simulink model "nav_sliding"  (R2022b)
settings: Solver=FixedStepAuto  StartTime=0.0  StopTime=10.0  FixedStep=0.01  RelTol=1e-3
values from neighbouring files (symbols this model uses):
  aR = diag([ar; ap; ay])    [main_flock3.m]    (also in main_flock4.m; main_sliding.m)
  Att_1 = [2 -2 -15]    [main_sliding.m]
  K1 = diag([k111; k122; k133])    [main_flock3.m]    (also in main_flock4.m; main_sliding.m)
  K2 = diag([k211; k222; k233])    [main_flock3.m]    (also in main_flock4.m; main_sliding.m)
  Ki = diag([Ki1; Ki2; Ki3])    [main_flock3.m]    (also in main_flock4.m; main_sliding.m)
  lam = diag([lam1; lam2; lam3])    [main_flock3.m]    (also in main_flock4.m; main_sliding.m)
  X0_1 = [P01 dP01 om01]    [main_flock3.m]    (also in main_flock4.m; main_sliding.m = [P0 dP0 om0])
undefined symbols (not defined in the file or in its folder): A_Euler
libraries: aerosimlib x1
settings Model: Creator=root  LastModifiedBy=jonatan_alvarez
settings SolverCC: AlgebraicLoopSolver=TrustRegion
settings DataIOCC: ReturnWorkspaceOutputs=off
settings DebuggingCC: UnconnectedInputMsg=warning  UnconnectedOutputMsg=warning  UnconnectedLineMsg=warning  SFMachineParentedDataDiag=warning  ArithmeticOperatorsInVariantConditions=warning
settings ModelReferenceCC: EnableRefExpFcnMdlSchedulingChecks=on
settings SFSimCC: CustomCodeUndefinedFunction=UseInterfaceOnly

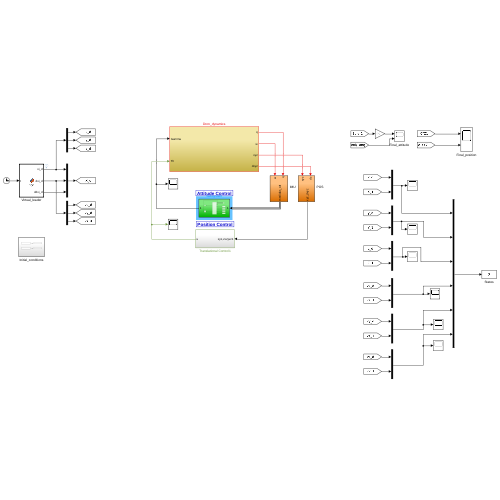
[thumbnail: Simulink's stored preview of the top-level diagram]
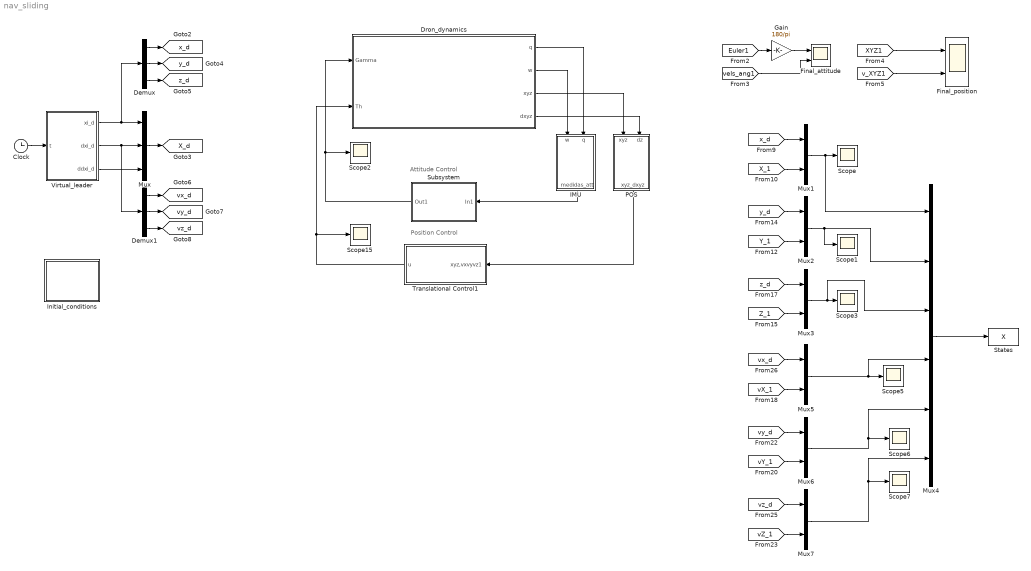
== system nav_sliding ==
  note: Position Control
  note: Attitude Control
  Clock : Clock
  Demux : Demux  Outputs=3
  Demux1 : Demux  Outputs=3
  Dron_dynamics : Subsystem
  Final_attitude : Scope  NumInputPorts=2
  Final_position : Scope  NumInputPorts=2
  Gain : Gain  Gain=180/pi
  "IMU " : Subsystem
  Initial_conditions : Subsystem
  Mux : Mux  Inputs=3
  Mux{1..3,5..7} (6 alike) : Mux  Inputs=2
  Mux4 : Mux  Inputs=6
  "POS " : Subsystem
  Scope{,1..3,5..7,15} (8 alike) : Scope
  States : ToWorkspace  VariableName=X  SampleTime=-1
  Subsystem : Subsystem
  Translational Control1 : Subsystem
  Virtual_leader : MATLAB Function  TreatAsAtomicUnit=on
  tag scope: X_d=global, vx_d=global, vy_d=global, vz_d=global, x_d=global, y_d=global, z_d=global
  wires:
  [vels_ang1] -> Final_attitude/2
  [v_XYZ1] -> Final_position/2
  Gain/1 -> Final_attitude/1
  [XYZ1] -> Final_position/1
  [Euler1] -> Gain/1
  Dron_dynamics/2(w) -> "IMU "/1(w)
  Dron_dynamics/4(dxyz) -> "POS "/2(dz)
  Mux/1 -> [X_d]
  Virtual_leader/3(ddxi_d) -> Mux/3
  Dron_dynamics/1(q) -> "IMU "/2(q)
  Subsystem/1(Out1) -> Scope2/1, Dron_dynamics/1(Gamma)
  Dron_dynamics/3(xyz) -> "POS "/1(xyz)
  "POS "/1(xyz_dxyz) -> Translational Control1/1(xyz,vxvyvz1)
  Translational Control1/1(u) -> Scope15/1, Dron_dynamics/2(Th)
  "IMU "/1(medidas_att) -> Subsystem/1(In1)
  Virtual_leader/1(xi_d) -> Demux/1, Mux/1
  Demux/1 -> [x_d]
  Demux/2 -> [y_d]
  Demux/3 -> [z_d]
  [x_d] -> Mux1/1
  [X_1] -> Mux1/2
  Mux2/1 -> Mux4/2, Scope1/1
  [Y_1] -> Mux2/2
  [y_d] -> Mux2/1
  [z_d] -> Mux3/1
  [Z_1] -> Mux3/2
  Mux3/1 -> Mux4/3, Scope3/1
  Mux4/1 -> States/1
  Mux1/1 -> Mux4/1, Scope/1
  Demux1/3 -> [vz_d]
  Demux1/2 -> [vy_d]
  Demux1/1 -> [vx_d]
  Virtual_leader/2(dxi_d) -> Demux1/1, Mux/2
  [vZ_1] -> Mux7/2
  [vz_d] -> Mux7/1
  [vy_d] -> Mux6/1
  [vY_1] -> Mux6/2
  [vX_1] -> Mux5/2
  [vx_d] -> Mux5/1
  Mux5/1 -> Scope5/1, Mux4/4
  Mux6/1 -> Scope6/1, Mux4/5
  Mux7/1 -> Scope7/1, Mux4/6
  Clock/1 -> Virtual_leader/1(t)

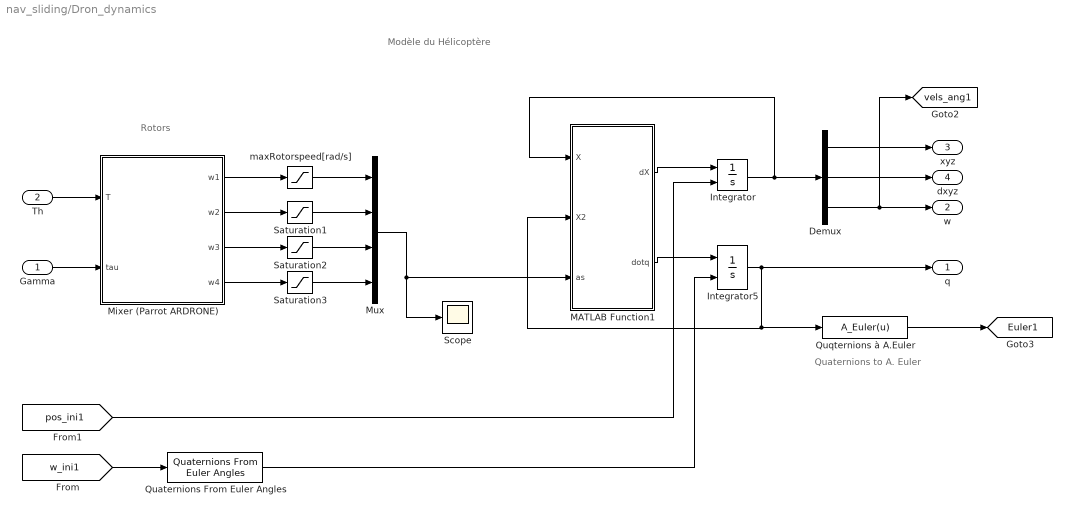
== system nav_sliding/Dron_dynamics ==
  note: Modèle du Hélicoptère
  note: Rotors
  note: Quaternions to A. Euler
  Gamma : Inport
  Th : Inport  Port=2
  Demux : Demux  Outputs=3
  Integrator : Integrator  InitialConditionSource=external
  Integrator5 : Integrator  InitialConditionSource=external  InitialCondition=[1 0 0 0]
  MATLAB Function1 : MATLAB Function  TreatAsAtomicUnit=on
  Mixer (Parrot ARDRONE) : MATLAB Function  TreatAsAtomicUnit=on
  Mux : Mux
  Quaternions From Euler Angles : aerosimlib/Transformations/Quaternions From Euler Angles
  Quqternions à A.Euler : MATLABFcn  MATLABFcn=A_Euler(u)  OutputDimensions=3
  Saturation1 : Saturate  UpperLimit=1100  LowerLimit=5
  Saturation2 : Saturate  UpperLimit=1100  LowerLimit=5
  Saturation3 : Saturate  UpperLimit=1100  LowerLimit=5
  Scope : Scope
  maxRotorspeed[rad/s] : Saturate  UpperLimit=1100  LowerLimit=5
  q : Outport  VectorParamsAs1DForOutWhenUnconnected=off
  w : Outport  Port=2  VectorParamsAs1DForOutWhenUnconnected=off
  xyz : Outport  Port=3  VectorParamsAs1DForOutWhenUnconnected=off
  dxyz : Outport  Port=4  VectorParamsAs1DForOutWhenUnconnected=off
  tag scope: Euler1=global, vels_ang1=global
  wires:
  [w_ini1] -> Quaternions From Euler Angles/1
  Quqternions à A.Euler/1 -> [Euler1]
  Mixer (Parrot ARDRONE)/4(w4) -> Saturation3/1
  Saturation1/1 -> Mux/2
  Mixer (Parrot ARDRONE)/2(w2) -> Saturation1/1
  Mixer (Parrot ARDRONE)/1(w1) -> maxRotorspeed[rad/s]/1
  maxRotorspeed[rad/s]/1 -> Mux/1
  Saturation3/1 -> Mux/4
  Saturation2/1 -> Mux/3
  Mixer (Parrot ARDRONE)/3(w3) -> Saturation2/1
  Mux/1 -> Scope/1, MATLAB Function1/3(as)
  Integrator5/1 -> MATLAB Function1/2(X2), Quqternions à A.Euler/1, q/1
  MATLAB Function1/1(dX) -> Integrator/1
  MATLAB Function1/2(dotq) -> Integrator5/1
  Quaternions From Euler Angles/1 -> Integrator5/2
  Integrator/1 -> Demux/1, MATLAB Function1/1(X)
  Gamma/1 -> Mixer (Parrot ARDRONE)/2(tau)
  [pos_ini1] -> Integrator/2
  Demux/3 -> [vels_ang1], w/1
  Demux/1 -> xyz/1
  Demux/2 -> dxyz/1
  Th/1 -> Mixer (Parrot ARDRONE)/1(T)

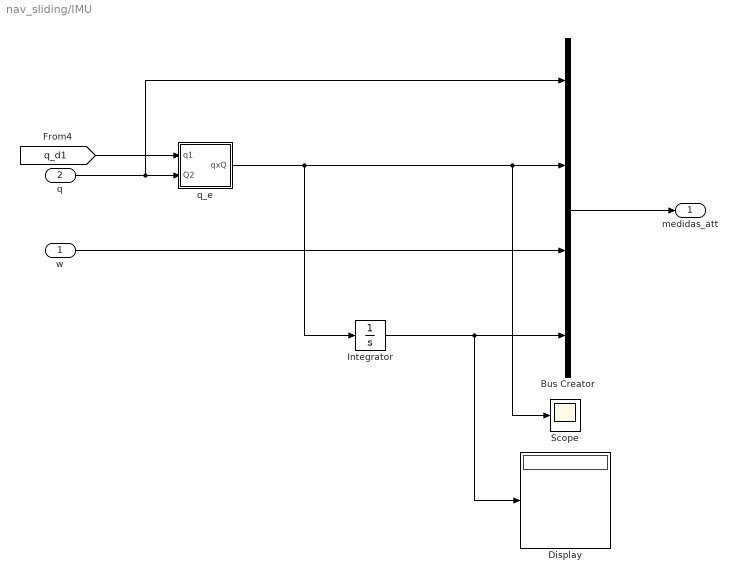
== system nav_sliding/IMU  ==
  w : Inport
  q : Inport  Port=2
  Bus Creator : BusCreator  Inputs=4
  Display : Display
  Integrator : Integrator
  Scope : Scope
  q_e : Subsystem
  medidas_att : Outport  VectorParamsAs1DForOutWhenUnconnected=off
  wires:
  [q_d1] -> q_e/1(q1)
  q/1 -> Bus Creator/1, q_e/2(Q2)
  w/1 -> Bus Creator/3
  Integrator/1 -> Display/1, Bus Creator/4
  Bus Creator/1 -> medidas_att/1
  q_e/1(qxQ) -> Integrator/1, Scope/1, Bus Creator/2

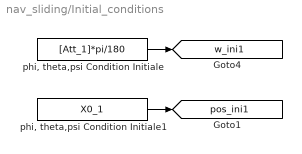
== system nav_sliding/Initial_conditions ==
  "phi, theta,psi Condition Initiale" : Constant  Value=[Att_1]*pi/180
  "phi, theta,psi Condition Initiale1" : Constant  Value=X0_1
  tag scope: pos_ini1=global, w_ini1=global
  wires:
  "phi, theta,psi Condition Initiale1"/1 -> [pos_ini1]
  "phi, theta,psi Condition Initiale"/1 -> [w_ini1]

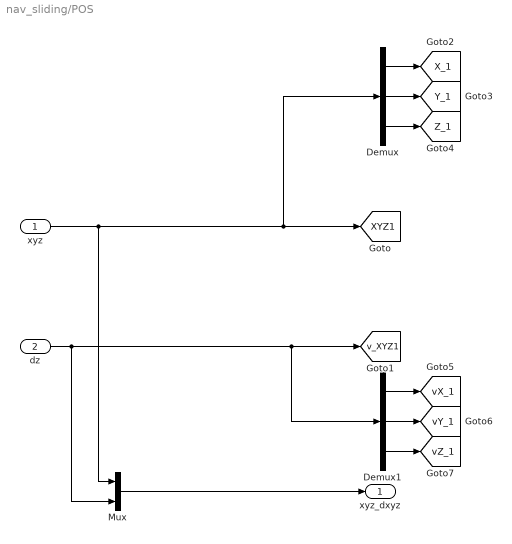
== system nav_sliding/POS  ==
  xyz : Inport
  dz : Inport  Port=2
  Demux : Demux  Outputs=3
  Demux1 : Demux  Outputs=3
  Mux : Mux  Inputs=2
  xyz_dxyz : Outport  VectorParamsAs1DForOutWhenUnconnected=off
  tag scope: XYZ1=global, X_1=global, Y_1=global, Z_1=global, vX_1=global, vY_1=global, vZ_1=global, v_XYZ1=global
  wires:
  xyz/1 -> Mux/1, Demux/1, [XYZ1]
  dz/1 -> Demux1/1, [v_XYZ1], Mux/2
  Demux/1 -> [X_1]
  Demux/2 -> [Y_1]
  Demux/3 -> [Z_1]
  Mux/1 -> xyz_dxyz/1
  Demux1/3 -> [vZ_1]
  Demux1/2 -> [vY_1]
  Demux1/1 -> [vX_1]

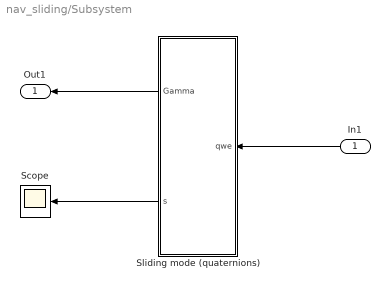
== system nav_sliding/Subsystem ==
  In1 : Inport
  Scope : Scope
  Sliding mode (quaternions) : MATLAB Function  Description=Integral quaternion Sliding mode control  TreatAsAtomicUnit=on
  Out1 : Outport  VectorParamsAs1DForOutWhenUnconnected=off
  wires:
  In1/1 -> Sliding mode (quaternions)/1(qwe)
  Sliding mode (quaternions)/1(Gamma) -> Out1/1
  Sliding mode (quaternions)/2(s) -> Scope/1

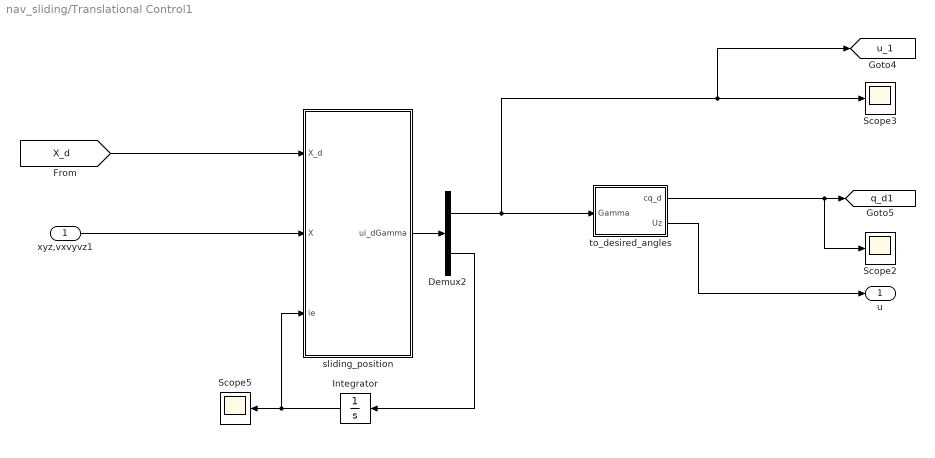
== system nav_sliding/Translational Control1 ==
  xyz,vxvyvz1 : Inport
  Demux2 : Demux  Outputs=2
  Integrator : Integrator
  Scope2 : Scope
  Scope3 : Scope
  Scope5 : Scope
  sliding_position : MATLAB Function  TreatAsAtomicUnit=on
  to_desired_angles : MATLAB Function  TreatAsAtomicUnit=on
  u : Outport  VectorParamsAs1DForOutWhenUnconnected=off
  tag scope: q_d1=global, u_1=global
  wires:
  sliding_position/1(ui_dGamma) -> Demux2/1
  to_desired_angles/2(Uz) -> u/1
  to_desired_angles/1(cq_d) -> Scope2/1, [q_d1]
  [X_d] -> sliding_position/1(X_d)
  xyz,vxvyvz1/1 -> sliding_position/2(X)
  Integrator/1 -> Scope5/1, sliding_position/3(ie)
  Demux2/2 -> Integrator/1
  Demux2/1 -> [u_1], Scope3/1, to_desired_angles/1(Gamma)

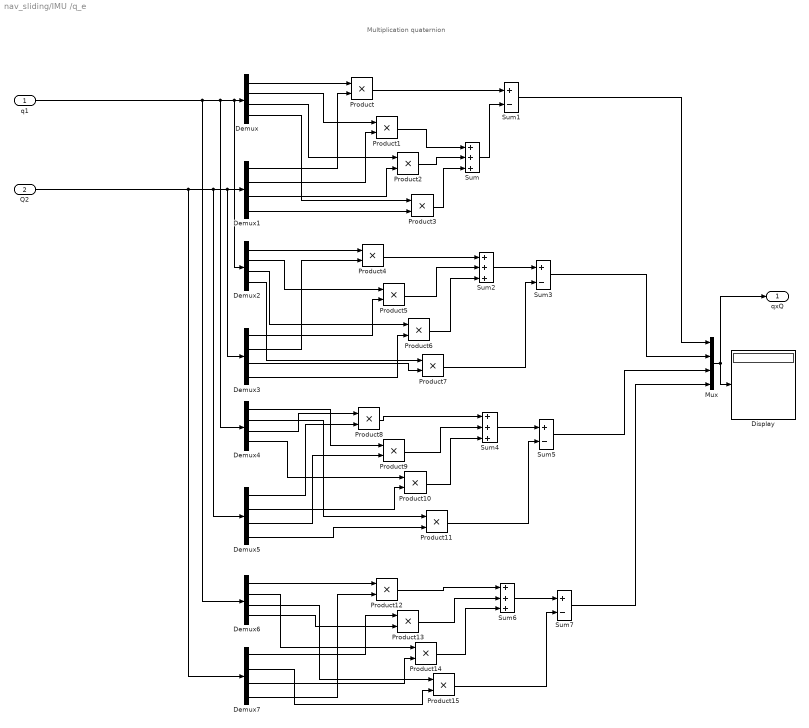
== system nav_sliding/IMU /q_e ==
  note: Multiplication quaternion
  q1 : Inport
  Q2 : Inport  Port=2
  Demux{,1..7} (8 alike) : Demux
  Display : Display
  Mux : Mux
  Product{,1..15} (16 alike) : Product  RndMeth=Zero
  Sum{,2,4,6} (4 alike) : Sum  Inputs=+++
  Sum{1,3,5,7} (4 alike) : Sum  Inputs=+-
  qxQ : Outport  VectorParamsAs1DForOutWhenUnconnected=off
  wires:
  q1/1 -> Demux/1, Demux2/1, Demux4/1, Demux6/1
  Q2/1 -> Demux1/1, Demux3/1, Demux5/1, Demux7/1
  Demux/1 -> Product/1
  Demux1/1 -> Product/2
  Demux/2 -> Product1/1
  Demux1/2 -> Product1/2
  Demux/3 -> Product2/1
  Demux1/3 -> Product2/2
  Demux/4 -> Product3/1
  Demux1/4 -> Product3/2
  Product1/1 -> Sum/1
  Product2/1 -> Sum/2
  Product3/1 -> Sum/3
  Sum/1 -> Sum1/2
  Product/1 -> Sum1/1
  Demux2/1 -> Product4/1
  Demux3/2 -> Product4/2
  Demux2/2 -> Product5/1
  Demux3/1 -> Product5/2
  Demux2/3 -> Product6/1
  Demux3/4 -> Product6/2
  Demux2/4 -> Product7/1
  Demux3/3 -> Product7/2
  Product4/1 -> Sum2/1
  Product5/1 -> Sum2/2
  Product6/1 -> Sum2/3
  Sum2/1 -> Sum3/1
  Product7/1 -> Sum3/2
  Demux4/3 -> Product8/1
  Demux5/1 -> Product8/2
  Demux4/1 -> Product9/1
  Demux5/3 -> Product9/2
  Demux4/4 -> Product10/1
  Demux5/2 -> Product10/2
  Demux5/4 -> Product11/2
  Demux4/2 -> Product11/1
  Sum4/1 -> Sum5/1
  Product11/1 -> Sum5/2
  Product8/1 -> Sum4/1
  Product9/1 -> Sum4/2
  Product10/1 -> Sum4/3
  Demux6/1 -> Product12/1
  Demux7/1 -> Product13/1
  Demux6/2 -> Product14/1
  Demux7/4 -> Product12/2
  Demux6/4 -> Product13/2
  Demux7/3 -> Product14/2
  Demux6/3 -> Product15/1
  Demux7/2 -> Product15/2
  Sum6/1 -> Sum7/1
  Product15/1 -> Sum7/2
  Product12/1 -> Sum6/1
  Product13/1 -> Sum6/2
  Product14/1 -> Sum6/3
  Sum1/1 -> Mux/1
  Sum3/1 -> Mux/2
  Sum5/1 -> Mux/3
  Sum7/1 -> Mux/4
  Mux/1 -> Display/1, qxQ/1

== matlab function nav_sliding/Dron_dynamics/Mixer (Parrot ARDRONE) ==
  data: T input; w1 output size=1; tau input; w2 output size=1; w3 output size=1; w4 output size=1
function [w1,w2,w3,w4]   = fcn(T, tau)
%#codegen
tau_phi = tau(1); 
tau_the = tau(2); 
tau_psi = tau(3);

% This values vary in fonction of the geometry of the drone 
b= 4.06e-6;
d= 7.5e-7;
l= (0.2)*(sin(pi/4));

%Parrot AR-DRONE 
uT = T/b; 
uphi = (sqrt(2)*tau_phi)/(b*l);  
uthe = (sqrt(2)*tau_the)/(b*l);
upsi = tau_psi/(d*l);

%Mix by Motors
mixM1 = uT+uphi-uthe+upsi;  %uT + for all mixM
mixM2 = uT-uphi-uthe-upsi; 
mixM3 = uT-uphi+uthe+upsi; 
mixM4 = uT+uphi+uthe-upsi;

%rotors speeds [rads/s]
w1= sign(mixM1)*sqrt(abs((1/4)*mixM1));
w2= sign(mixM2)*sqrt(abs((1/4)*mixM2));
w3= sign(mixM3)*sqrt(abs((1/4)*mixM3));
w4= sign(mixM4)*sqrt(abs((1/4)*mixM4));

== matlab function nav_sliding/Virtual_leader ==
  data: t input; xi_d output; dxi_d output; ddxi_d output
function [xi_d, dxi_d, ddxi_d]  = fcn(t)
%#codegen

f=1/14;    %freq in Hz
radius=2;   %radius in meters
f2 = 1/35;
radius2 = 1;
sel=1;      %inputs or parameters dont work! only local vars ...

if sel == 1
    if t < 15
       xd     =  0;
       xdotd  =  0;
       xddotd =  0;   
    
       yd     = 0;
       ydotd  = 0;
       yddotd = 0;
    
       zd     = 2;  
       zdotd  = 0; 
       zddotd = 0;
    
       xi_d =[xd; yd; zd];
       dxi_d=[xdotd; ydotd; zdotd]; 
       ddxi_d = [xddotd; yddotd; zddotd];
    elseif t < 30
        xd     =  1.5;
        xdotd  =  0;
        xddotd =  0;   
    
        yd     = -1;
        ydotd  = 0;
        yddotd = 0;
    
        zd     = 2;  
        zdotd  = 0; 
        zddotd = 0;
    
        xi_d =[xd; yd; zd];
        dxi_d=[xdotd; ydotd; zdotd]; 
        ddxi_d = [xddotd; yddotd; zddotd];
    else
       scale = 6 / (3 - cos(2*f*t));
    
       xd     = scale * cos(f*t);
       xdotd  = (7*f*(sin(f*t)*(cos(2*f*t)-3)-2*sin(2*f*t)*cos(f*t))) / (3-cos(2*f*t))^2;  
       xddotd = 0;   %xdd;
    
       yd     = scale * sin(2*f*t) / 2;
       ydotd  = -(7*f*((sin(2*f*t)^2 + cos(2*f*t)^2) - 3*cos(2*f*t))) / (3-cos(2*f*t))^2;
       yddotd = 0;  %ydd;
    
       zd     = radius2*sin(2*pi*f2*t) + 4;
       zdotd  = radius2*2*pi*f2*cos(2*pi*f2*t);
       zddotd = -radius2*4*pi^2*f2^2*sin(2*pi*f2*t);
    
       xi_d =[xd; yd; zd];
       dxi_d=[xdotd; ydotd; zdotd];
       ddxi_d = [xddotd; yddotd; zddotd];
    end
end

 if(sel==2)
     xd     =  0.5;
     xdotd  =  0;
     xddotd =  0;   
     
     yd     = 0.5;
     ydotd  = 0;
     yddotd = 0;
     
     zd     = 1.5;  
     zdotd  = 0; 
     zddotd = 0;
     
     xi_d =[xd; yd; zd];
     dxi_d=[xdotd; ydotd; zdotd]; 
     ddxi_d = [xddotd; yddotd; zddotd];
 end

== matlab function nav_sliding/Subsystem/Sliding mode (quaternions) ==
  data: qwe input; Gamma output; lam parameter; Ki parameter; K1 parameter; K2 parameter; aR parameter; s output
function [Gamma, s]  = fcn(qwe, lam, Ki, K1, K2, aR)

%Rotorcraft dimensions and parameters
Ix = 7.5e-3;
Iy = 7.5e-3;
Iz = 1.3e-2;

%Inertia
Ii=[Ix 0 0; 0 Iy 0; 0 0 Iz];

%Separation of rotational velocity and quaternion error in its components
qe = qwe(5:8);
qe1 = qe(1);
qe2 = qe(2);
qe3 = qe(3);
qe4 = qe(4);
qev = [qe2; qe3; qe4];

w = qwe(9:11);

iqe = qwe(12:15);
i_qe = [iqe(2); iqe(3); iqe(4)];

%Desired rotational velocity
wd = [0;0;0];

dwd = [0;0;0];

%Rotational velocity error in Euler
we = w - wd;
we1 = we(1);
we2 = we(2);
we3 = we(3);

%Quaternion error (derivative)
dqe0 = 0.5*(-we1*qe2 - we2*qe3 - we3*qe4);
dqe1 = 0.5*(we1*qe1 + we3*qe3 - we2*qe4);
dqe2 = 0.5*(we2*qe1 - we3*qe2 + we1*qe4);
dqe3 = 0.5*(we3*qe1 + we2*qe2 - we1*qe3);
dqe = [dqe1; dqe2; dqe3];

%Identity matrix
I3 = [1 0 0;
      0 1 0;
      0 0 1];
%Skew symmetrix matrix of vector part of the quaternion
sqev = [0 -qe4 qe3;
       qe4 0 -qe2;
       -qe3 qe2 0];
%ROTAION MATRIX: Given in Euler-Rodrigues formula
Re = (qe1^2 - qev'*qev)*I3 + 2*(qev*qev') - 2*qe1*sqev;

s = Ii*we + lam*qev + Ki*i_qe;

prod = cross(we,Re'*wd);

u = -lam*dqe - Ki*qev -Ii*(prod - Re'*dwd) + cross(w,Ii*w);       %Ks*qev

%Integral SMC 
Gamma = u - K1*tanh(inv(aR)*s) - K2*s;

== matlab function nav_sliding/Translational Control1/sliding_position ==
  data: X_d input; ui_dGamma output; X input; ie input; KP parameter
function ui_dGamma = fcn(X_d, X, ie, KP)

%Rotorcraft dimensions and parameters
m = 0.65;   
g = 9.81;

%Control gains 
Kx = KP(1); Ky = KP(2); Kz = KP(3);
Kdx = KP(4); Kdy = KP(5); Kdz = KP(6);
Kix = KP(7); Kiy = KP(8); Kiz = KP(9);

%Separation of desired and actual positions, velocities ans accelerations in their components
X_l = X_d(1:9); 
xl = X_l(1);    vxl = X_l(4);   ddxd = X_l(7);   
yl = X_l(2);    vyl = X_l(5);   ddyd = X_l(8);
zl = X_l(3);    vzl = X_l(6);   ddzd = X_l(9);

X_a = X(1:6);
xac = X_a(1);     vxac = X_a(4);
yac = X_a(2);     vyac = X_a(5);
zac = X_a(3);     vzac = X_a(6);

%Integral of the error
ieX = ie(1:3);
iex = ieX(1);
iey = ieX(2);
iez = ieX(3);

%Errors definition (position and velocity)
ex = xl - xac;    evx = vxl - vxac;
ey = yl - yac;    evy = vyl - vyac;
ez = zl - zac;    evz = vzl - vzac;

%First part of the control u_o
u_ox = Kx*ex + Kdx*evx + Kix*iex;
u_oy = Ky*ey + Kdy*evy + Kiy*iey;
u_oz = Kz*ez + Kdz*evz + Kiz*iez;

ui_dGamma = [u_ox;u_oy;u_oz;ex;ey;ez];

== matlab function nav_sliding/Translational Control1/to_desired_angles ==
  data: Gamma input; cq_d output; Uz output
function [cq_d,Uz] = fcn(Gamma)

%Physical parameters
m = 0.65;
g = 9.81;

%Control signals separation
gamma = Gamma(1:3);
gamma1 = gamma(1);
gamma2 = gamma(2);
gamma3 = gamma(3);

%Desired Phi, theta, trust
psi = 0*pi/180;

phi = atan(gamma2/(gamma3+g));

theta = asin(-gamma1/(sqrt(gamma1^2+gamma2^2+(gamma3+g)^2)));

Uz = m*sqrt((gamma1)^2+(gamma2)^2+(gamma3+g)^2);

%Conversion to quaternions
q0 = cos(psi/2)*cos(theta/2)*cos(phi/2) + sin(psi/2)*sin(theta/2)*sin(phi/2);
q1 = cos(psi/2)*cos(theta/2)*sin(phi/2) - sin(psi/2)*sin(theta/2)*cos(phi/2);
q2 = cos(psi/2)*sin(theta/2)*cos(phi/2) + sin(psi/2)*cos(theta/2)*sin(phi/2);
q3 = sin(psi/2)*cos(theta/2)*cos(phi/2) - cos(psi/2)*sin(theta/2)*sin(phi/2);

cq_d = [q0;
        -q1;
        -q2;
        -q3];

== matlab function nav_sliding/Dron_dynamics/MATLAB Function1 ==
  data: X input; dX output; X2 input; dotq output; as input
function [dX,dotq] = fcn(X, X2, as)
% Jonatan Alvarez / October 2021
% Rotorcraft 3D Model (based on the quaternion parametrization) 

%Rotorcraft dimensions and parameters
m=0.65;   
g = 9.81;
Ix = 7.5e-3;
Iy = 7.5e-3;
Iz = 1.3e-2;
e  = 4.06e-6;
d  = 7.5e-7;
l  = (0.2)*(sin(pi/4));

%Inertia
Ii=[Ix 0 0; 0 Iy 0; 0 0 Iz];

%Extraction of data
x = X(1:3);
dx = X(4:6);
om = X(7:9); %Angular velocity

%Wind


%Separation of the angular velocity and quaternions in its components
om1 = om(1);
om2 = om(2);
om3 = om(3);

q = X2(1:4);
q1 = q(1);
q2 = q(2);
q3 = q(3);
q4 = q(4);
qv = [q2;q3;q4];

%EXTRACTION OF ROTOR SPEEDS AND FORCES COMPUTATION
u = as(1:4);
%Motor forces (e3)
f1= e*u(1)^2; f2=e*u(2)^2;  f3=e*u(3)^2; f4=e*u(4)^2; % rotors' blades lift forces
f1d = d*u(1)^2; f2d=d*u(2)^2;  f3d=d*u(3)^2; f4d=d*u(4)^2; %rotors' blades drag forces
%Torques
tau_phi = (1/sqrt(2))*l*(f1-f2-f3+f4) ;
tau_the = (1/sqrt(2))*l*(-f1-f2+f3+f4);
tau_psi = l*(f1d-f2d+f3d-f4d);
%MAIN Thrust and Torque vectors
Th =[0;0;f1+f2+f3+f4];
F = [tau_phi;tau_the;tau_psi];

%ROTATIONAL MOTION
%Quaternions
dq0 = 0.5*(-om1*q2 - om2*q3 - om3*q4);
dq1 = 0.5*(om1*q1 + om3*q3 - om2*q4);
dq2 = 0.5*(om2*q1 - om3*q2 + om1*q4);
dq3 = 0.5*(om3*q1 + om2*q2 - om1*q3);
%Attitude kinematics in quaternions
dotq = [dq0;dq1;dq2;dq3];  
%Attitude dynamics
dW =  inv(Ii)*( - cross(om,Ii*om) + F);

%TRANSLATIONAL MOTION
%Identity matrix
I3 = [1 0 0;
      0 1 0;
      0 0 1];
%Skew symmetrix matrix of vector part of the quaternion
sqv = [0 -q4 q3;
       q4 0 -q2;
       -q3 q2 0];
%Rotation matrix: given in Euler-Rodrigues formula
R = (q1^2 - qv'*qv)*I3 + 2*(qv*qv') - 2*q1*sqv;
%R = I3 - 2*q1*(sqv) + 2*(sqv)^2;
%Mass matrix
M_xi=[m  0  0;
      0  m  0;
      0  0  m];
%Vector fo Gravitational terms and thrust
G_xi=[0;0;m*g];
%Th = [0;0;T];
%Linear dynamics
Ddx =  inv(M_xi)*( -G_xi + R*Th);  % +fa

%Final vector
dX = [dx;Ddx;dW];
